simulink model "ph_openloop"  (R2021a)
settings: Solver=VariableStepAuto  StartTime=0.0  StopTime=400  RelTol=1e-3
settings Model: Creator=USER  LastModifiedBy=USER

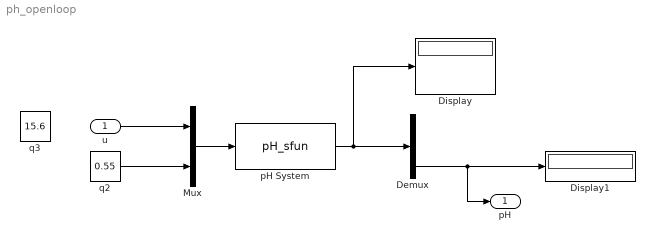
== system ph_openloop ==
  u : Inport
  Demux : Demux  Outputs=3
  Display : Display
  Display1 : Display
  Mux : Mux  Inputs=2
  pH System : S-Function  FunctionName=pH_sfun  SFunctionDeploymentMode=off  EnableBusSupport=off
  q2 : Constant  Value=0.55
  q3 : Constant  Value=15.6
  pH : Outport
  wires:
  Mux/1 -> pH System/1
  pH System/1 -> Demux/1, Display/1
  u/1 -> Mux/1
  q2/1 -> Mux/2
  Demux/3 -> Display1/1, pH/1
